simulink model "singlephasecycloconverter"  (Simulink 7.3)
settings: Solver=ode23tb  StartTime=0.0  StopTime=0.06  MaxStep=1e-5  RelTol=1e-3
libraries: powerlib x15, simulink x1
settings Model: Creator=viswam  LastModifiedBy=viswam
settings SolverCC: InitialStep=1e-6
settings OptimizationCC: InitFltsAndDblsToZero=on
settings DebuggingCC: SaveWithParameterizedLinksMsg=none  SignalResolutionControl=TryResolveAllWithWarning  MultiTaskDSMMsg=warning  MultiTaskCondExecSysMsg=none
settings RTWCC: IncludeERTFirstTime=on
settings GRTTargetCC: TargetFcnLib=ansi_tfl_tmw.mat

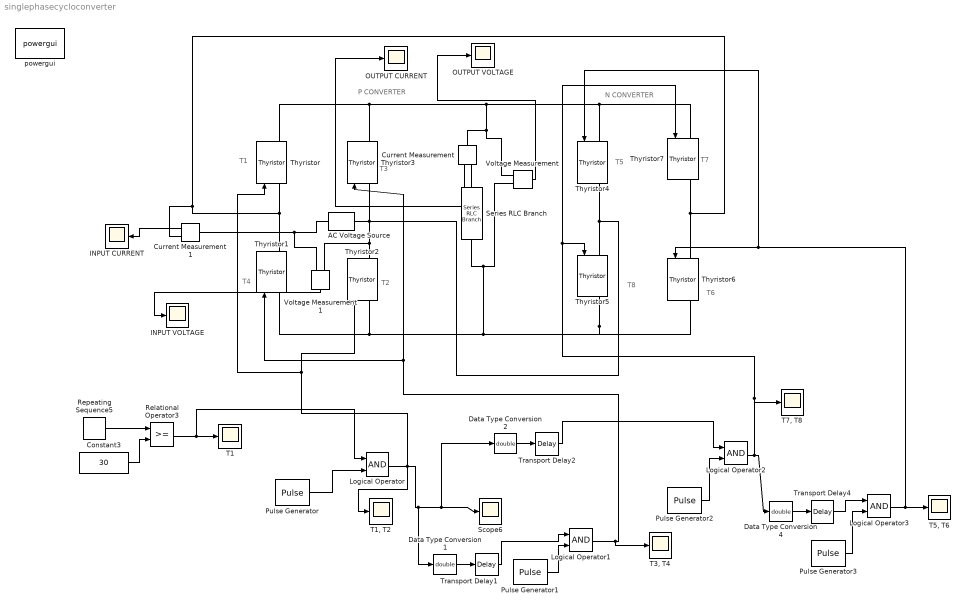
== system singlephasecycloconverter ==
  note: T1
  note: T2
  note: T3
  note: T4
  note: T5
  note: T6
  note: T7
  note: T8
  note: P CONVERTER
  note: N CONVERTER
  AC Voltage Source : powerlib/Electrical Sources/AC Voltage Source  DialogController=POWERSYS.PowerSysDialog  SystemSampleTime=-1  Amplitude=325.26  Phase=0  Frequency=50  SampleTime=0  Measurements=None
  Constant3 : Constant  Value=30  OutDataType=sfix(16)  OutScaling=2^0
  Current Measurement : powerlib/Measurements/Current Measurement  DialogController=POWERSYS.PowerSysDialog  SystemSampleTime=-1  PhasorSimulation=off  OutputType=Complex  PSBequivalent=0
  Current Measurement1 : powerlib/Measurements/Current Measurement  DialogController=POWERSYS.PowerSysDialog  SystemSampleTime=-1  PhasorSimulation=off  OutputType=Complex  PSBequivalent=0
  Data Type Conversion1 : DataTypeConversion  OutDataTypeMode=double  OutDataType=sfix(16)  OutScaling=2^0  OutDataTypeStr=double
  Data Type Conversion2 : DataTypeConversion  OutDataTypeMode=double  OutDataType=sfix(16)  OutScaling=2^0  OutDataTypeStr=double
  Data Type Conversion4 : DataTypeConversion  OutDataTypeMode=double  OutDataType=sfix(16)  OutScaling=2^0  OutDataTypeStr=double
  INPUT CURRENT : Scope
      settings: TimeRange=0.1  YMin=-50  YMax=10  SaveName=inpucurrent  SampleInput=on  SampleTime=1e-5
  INPUT VOLTAGE : Scope
      settings: TimeRange=0.1  YMin=-50  YMax=10  SaveName=inputvoltage  SampleInput=on  SampleTime=1e-5
  Logical Operator{,1..3} (4 alike) : Logic  AllPortsSameDT=off  OutDataTypeMode=boolean  OutDataTypeStr=boolean
  OUTPUT CURRENT : Scope
      settings: TimeRange=0.1  YMin=-50  YMax=10  SaveName=outputcurrent  SampleInput=on  SampleTime=1e-5
  OUTPUT VOLTAGE : Scope
      settings: TimeRange=0.1  YMin=-100  YMax=100  SaveName=outputvoltage  SampleInput=on  SampleTime=1e-5
  Pulse Generator : DiscretePulseGenerator  PulseType=Time based  Amplitude=1  Period=0.06  PulseWidth=50  PhaseDelay=0  SampleTime=1
  Pulse Generator1 : DiscretePulseGenerator  PulseType=Time based  Amplitude=1  Period=0.06  PulseWidth=50  PhaseDelay=0  SampleTime=1
  Pulse Generator2 : DiscretePulseGenerator  PulseType=Time based  Amplitude=1  Period=0.06  PulseWidth=50  PhaseDelay=0.03  SampleTime=1
  Pulse Generator3 : DiscretePulseGenerator  PulseType=Time based  Amplitude=1  Period=0.06  PulseWidth=50  PhaseDelay=0.03  SampleTime=1
  Relational Operator3 : RelationalOperator  LogicOutDataTypeMode=boolean  OutDataTypeStr=boolean
  Repeating Sequence5 : simulink/Sources/Repeating Sequence  SystemSampleTime=-1  rep_seq_t=[0 0.01 0.01 0.02]  rep_seq_y=[0 180 0 0]
  Scope6 : Scope
      settings: SaveName=ScopeData6
  Series RLC Branch : powerlib/Elements/Series RLC Branch  DialogController=POWERSYS.PowerSysDialog  PhysicalDomain=powersysdomain  SubClassName=unknown  LeftPortType=p1  RightPortType=p1  LConnTagsString=__new0  RConnTagsString=__new0  BranchType=R  Resistance=10  Inductance=1e-3  SetiL0=off  InitialCurrent=0  Capacitance=1e-6  Setx0=off  InitialVoltage=0  Measurements=None
  T1 : Scope
      settings: SaveName=ScopeData5
  "T1, T2" : Scope
  "T3, T4" : Scope
  "T5, T6" : Scope
      settings: TimeRange=0.06  SaveName=ScopeData4
  "T7, T8" : Scope
      settings: SaveName=ScopeData2
  Thyristor{,1..7} (8 alike) : powerlib/Power Electronics/Thyristor  DialogController=POWERSYS.PowerSysDialog  SystemSampleTime=-1  Ron=0.001  Lon=0  Vf=0.8  IC=0  Rs=500  Cs=250e-9  Measurements=on
  Transport Delay1 : TransportDelay  DelayTime=0.01
  Transport Delay2 : TransportDelay  DelayTime=0.03
  Transport Delay4 : TransportDelay  DelayTime=0.01
  Voltage Measurement : powerlib/Measurements/Voltage Measurement  DialogController=POWERSYS.PowerSysDialog  SystemSampleTime=-1  PhasorSimulation=off  OutputType=Complex  PSBequivalent=0
  Voltage Measurement1 : powerlib/Measurements/Voltage Measurement  DialogController=POWERSYS.PowerSysDialog  SystemSampleTime=-1  PhasorSimulation=off  OutputType=Complex  PSBequivalent=0
  powergui : powerlib/powergui  Priority=1  SystemSampleTime=-1  SimulationMode=Continuous  SampleTime=50e-6  frequency=60  SPID=off  DisableSnubberDevices=off  DisableRonSwitches=off  DisableVfSwitches=off  SwTol=0  Interpol=off  frequencyindice=50  echomessages=off  HookPort=off  DisplayEquations=off  FunctionMessages=off  EnableUseOfTLC=off  x0status=blocks  RestoreLinks=warning  Frange=[0:2:500]  Ylog=off  Xlog=on  ShowGrid=off  save=off  variable=ZData  ZoomFFT=on  StartTime=0.0  cycles=1  DisplayStyle=1  fundamental=60  FreqAxis=off  MaxFrequency=1000  frequencyindicesteady=1  RmsSteady=1  display=off  Ts=0  methode=off
  wires:
  Data Type Conversion1/1 -> Transport Delay1/1
  Repeating Sequence5/1 -> Relational Operator3/1
  Constant3/1 -> Relational Operator3/2
  Relational Operator3/1 -> T1/1, Logical Operator/1
  Pulse Generator/1 -> Logical Operator/2
  Logical Operator/1 -> Data Type Conversion1/1, Scope6/1, Data Type Conversion2/1, Thyristor2/1, Thyristor/1, "T1, T2"/1
  Voltage Measurement/1 -> OUTPUT VOLTAGE/1
  Transport Delay1/1 -> Logical Operator1/1
  Pulse Generator1/1 -> Logical Operator1/2
  Logical Operator1/1 -> Thyristor3/1, Thyristor1/1, "T3, T4"/1
  Data Type Conversion2/1 -> Transport Delay2/1
  Transport Delay2/1 -> Logical Operator2/1
  Pulse Generator2/1 -> Logical Operator2/2
  Logical Operator2/1 -> Data Type Conversion4/1, Thyristor5/1, Thyristor7/1, "T7, T8"/1
  Data Type Conversion4/1 -> Transport Delay4/1
  Pulse Generator3/1 -> Logical Operator3/2
  Transport Delay4/1 -> Logical Operator3/1
  Logical Operator3/1 -> "T5, T6"/1, Thyristor6/1, Thyristor4/1
  Current Measurement/1 -> OUTPUT CURRENT/1
  Voltage Measurement1/1 -> INPUT VOLTAGE/1
  Current Measurement1/1 -> INPUT CURRENT/1
  connections:
  Thyristor2/LConn1 -- Thyristor1/LConn1 -- Voltage Measurement/LConn2 -- Series RLC Branch/RConn1 -- Thyristor6/RConn1 -- Thyristor5/RConn1
  Thyristor1/RConn1 -- Thyristor/LConn1 -- Thyristor6/LConn1 -- Thyristor7/RConn1 -- Current Measurement1/RConn1
  Thyristor3/LConn1 -- AC Voltage Source/LConn1 -- Thyristor5/LConn1 -- Thyristor4/RConn1 -- Thyristor2/RConn1 -- Voltage Measurement1/LConn2
  Thyristor7/LConn1 -- Thyristor4/LConn1 -- Thyristor/RConn1 -- Thyristor3/RConn1 -- Voltage Measurement/LConn1 -- Current Measurement/LConn1
  Current Measurement/RConn1 -- Series RLC Branch/LConn1
  AC Voltage Source/RConn1 -- Current Measurement1/LConn1 -- Voltage Measurement1/LConn1
